simulink model "learjet"  (Simulink 6.3)
settings: Solver=ode4  StartTime=0.0  StopTime=100.0  FixedStep=0.1  RelTol=1e-3
values from neighbouring files (symbols this model uses):
  bref = 34    [learjet_iterate_trim_hood.m]    (also in learjet_iterate_trim_student.m; learjetstudent.m)
  cbar = 27.3    [hw5_714.m]    (also in hw6_714.m = 7; learjet_iterate_trim_hood.m = 7.04; learjet_iterate_trim_student.m = 7.04; learjetstudent.m = 7.04)
  CD0 = .0431    (= 0.0431)    [learjet_iterate_trim_hood.m]    (also in learjet_iterate_trim_student.m; learjetstudent.m = 0.1635)
  CD0BAR = .01867    (= 0.01867)    [learjet_iterate_trim_hood.m]    (also in learjet_iterate_trim_student.m; learjetstudent.m)
  CDA = 1.06    [learjet_iterate_trim_hood.m]    (also in learjet_iterate_trim_student.m; learjetstudent.m)
  CDDE = 0    [learjet_iterate_trim_hood.m]    (also in learjet_iterate_trim_student.m; learjetstudent.m)
  CDDETAB = 0    [learjet_iterate_trim_hood.m]    (also in learjet_iterate_trim_student.m; learjetstudent.m)
  CDK = .18824    (= 0.18824)    [learjet_iterate_trim_hood.m]    (also in learjet_iterate_trim_student.m; learjetstudent.m)
  CL0 = 1.2    [learjet_iterate_trim_hood.m]    (also in learjet_iterate_trim_student.m; learjetstudent.m)
  CLA = 5.04    [learjet_iterate_trim_hood.m]    (also in learjet_iterate_trim_student.m; learjetstudent.m)
  CLADOTHAT = 1.6    [learjet_iterate_trim_hood.m]    (also in learjet_iterate_trim_student.m; learjetstudent.m)
  CLDE = .40    (= 0.4)    [learjet_iterate_trim_hood.m]    (also in learjet_iterate_trim_student.m; learjetstudent.m)
  CLDETAB = CLDE/6.    (= 0.0666666666667)    [learjet_iterate_trim_hood.m]    (also in learjet_iterate_trim_student.m; learjetstudent.m)
  CLQHAT = 4.1    [learjet_iterate_trim_hood.m]    (also in learjet_iterate_trim_student.m; learjetstudent.m)
  CM0 = .047    (= 0.047)    [learjet_iterate_trim_hood.m]    (also in learjet_iterate_trim_student.m; learjetstudent.m)
  CMA = -.66    (= -0.66)    [learjet_iterate_trim_hood.m]    (also in learjet_iterate_trim_student.m; learjetstudent.m)
  CMADOTHAT = -5.0    (= -5)    [learjet_iterate_trim_hood.m]    (also in learjet_iterate_trim_student.m; learjetstudent.m)
  CMDE = -0.98    [learjet_iterate_trim_hood.m]    (also in learjet_iterate_trim_student.m; learjetstudent.m)
  CMDETAB = CMDE/6    (= -0.163333333333)    [learjet_iterate_trim_hood.m]    (also in learjet_iterate_trim_student.m; learjetstudent.m)
  CMQHAT = -13.5    [learjet_iterate_trim_hood.m]    (also in learjet_iterate_trim_student.m; learjetstudent.m)
  cosit = cos(it)    [learjet_iterate_trim_hood.m]    (also in learjet_iterate_trim_student.m; learjetstudent.m)
  detrim = dehat*(180/pi)    [learjet_iterate_trim_hood.m]    (also in learjet_iterate_trim_student.m; learjetstudent.m = 0)
  dPMdT = 0    [learjet_iterate_trim_hood.m]    (also in learjet_iterate_trim_student.m; learjetstudent.m)
  hic = 0    [learjet_iterate_trim_hood.m]    (also in learjet_iterate_trim_student.m; learjetstudent.m)
  inertia_matrix = [Ixxb 0 -Ixzb; 0 Iyyb 0;Ixzb 0 Izzb]    [learjet_iterate_trim_hood.m]    (also in learjet_iterate_trim_student.m; learjetstudent.m)
  mass = Wt/g    (= 403.726708075)    [learjet_iterate_trim_hood.m]    (also in learjet_iterate_trim_student.m; learjetstudent.m)
  phiic = 0    [learjet_iterate_trim_hood.m]    (also in learjet_iterate_trim_student.m; learjetstudent.m)
  psiic = 0    [learjet_iterate_trim_hood.m]    (also in learjet_iterate_trim_student.m; learjetstudent.m)
  sinit = sin(it)    [learjet_iterate_trim_hood.m]    (also in learjet_iterate_trim_student.m; learjetstudent.m)
  Sref = 232    [learjet_iterate_trim_hood.m]    (also in learjet_iterate_trim_student.m; learjetstudent.m)
  thetaic = alpha    [learjet_iterate_trim_hood.m]    (also in learjet_iterate_trim_student.m; learjetstudent.m = 0.0698131700798)
  thrust = thrusthat    [learjet_iterate_trim_hood.m]    (also in learjet_iterate_trim_student.m; learjetstudent.m = 1000)
  U1 = 100:50:400    [hw5_714.m]    (also in hw6_714.m = 170; learjet_iterate_trim_hood.m = 170; learjet_iterate_trim_student.m = 170; learjetstudent.m = 170)
  Uic = U1*cos(alpha)    [learjet_iterate_trim_hood.m]    (also in learjet_iterate_trim_student.m; learjetstudent.m)
  Vic = 0    [learjet_iterate_trim_hood.m]    (also in learjet_iterate_trim_student.m; learjetstudent.m)
  Wic = U1*sin(alpha)    [learjet_iterate_trim_hood.m]    (also in learjet_iterate_trim_student.m; learjetstudent.m)
  Wt = 13000    [learjet_iterate_trim_hood.m]    (also in learjet_iterate_trim_student.m; learjetstudent.m)
libraries: aerospace x7
settings Model: LastModifiedBy=jsteck  BufferReuse=off  StrictBusMsg=None
settings DataIOCC: SignalLoggingName=sigsOut
settings OptimizationCC: BooleanDataType=off  OptimizeBlockIOStorage=off  BufferReuse=off  ExpressionFolding=off  LocalBlockOutputs=off
settings DebuggingCC: SolverPrmCheckMsg=none
settings HardwareCC: TargetUnknown=on

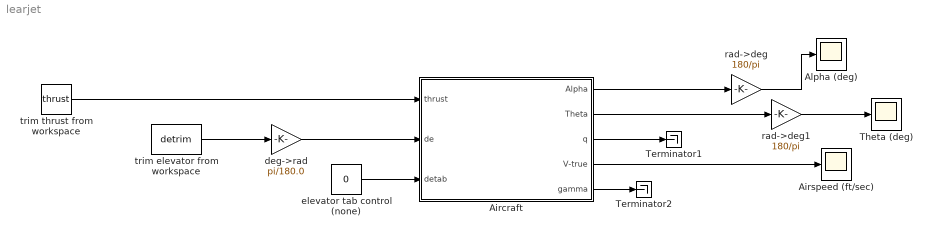
== system learjet ==
  Aircraft : Subsystem
  Airspeed (ft/sec) : Scope
      settings: TimeRange=100  YMin=100  YMax=200  SaveName=ScopeData4
  Alpha (deg) : Scope
      settings: TimeRange=100  YMin=0  YMax=8  SaveName=ScopeData3
  Terminator1 : Terminator
  Terminator2 : Terminator
  Theta (deg) : Scope
      settings: TimeRange=100  YMin=0  YMax=8  SaveName=ScopeData6
  deg->rad : Gain  Gain=pi/180.0  SaturateOnIntegerOverflow=on
  elevator tab control (none) : Constant  Value=0
  rad->deg : Gain  Gain=180/pi  SaturateOnIntegerOverflow=on
  rad->deg1 : Gain  Gain=180/pi  SaturateOnIntegerOverflow=on
  trim elevator from workspace : Constant  Value=detrim
  trim thrust from workspace : Constant  Value=thrust
  wires:
  elevator tab control (none)/1 -> Aircraft/3(detab)
  trim thrust from workspace/1 -> Aircraft/1(thrust)
  trim elevator from workspace/1 -> deg->rad/1
  Aircraft/1(Alpha) -> rad->deg/1
  Aircraft/4(V-true) -> Airspeed (ft/sec)/1
  Aircraft/2(Theta) -> rad->deg1/1
  Aircraft/3(q) -> Terminator1/1
  Aircraft/5(gamma) -> Terminator2/1
  deg->rad/1 -> Aircraft/2(de)
  rad->deg/1 -> Alpha (deg)/1
  rad->deg1/1 -> Theta (deg)/1

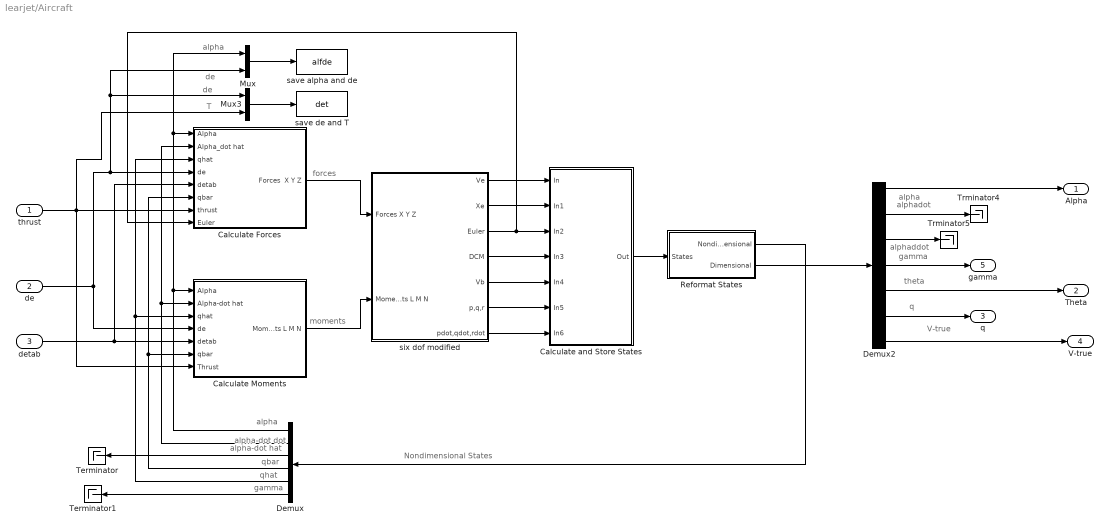
== system learjet/Aircraft ==
  note: Nondimensional States
  note: alpha
  note: alpha-dot hat
  note: gamma
  note: qbar
  note: forces
  note: moments
  note: de
  note: alpha
  note: de
  note: T
  note: alpha-dot dot
  note: qhat
  note: alpha
  note: alphadot
  note: alphaddot
  note: theta
  note: q
  note: gamma
  note: V-true
  thrust : Inport
  de : Inport  Port=2
  detab : Inport  Port=3
  Calculate Forces : Subsystem
  Calculate Moments : Subsystem
  Calculate and Store States : Subsystem
  Demux : Demux  Orientation=left  Outputs=6
  Demux2 : Demux  Outputs=7
  Mux : Mux  Inputs=2
  Mux3 : Mux  Inputs=2
  Reformat States : Subsystem
  Terminator : Terminator
  Terminator1 : Terminator
  Trminator4 : Terminator
  Trminator5 : Terminator
  save alpha and de : ToWorkspace  VariableName=alfde  SampleTime=-1  SaveFormat=Array
  save de and T : ToWorkspace  VariableName=det  SampleTime=-1  SaveFormat=Array
  six dof modified : Subsystem  AncestorBlock=aerospace/6DoF/Euler Angles  mask(6DoF Equations of Motion){xme_0=[0 0 hic], Vm_0=[Uic Vic Wic], eul_0=[phiic thetaic psiic], pm_0=[0 0 0], Mass=mass, Inertia=inertia_matrix}
      mask prompts: xme_0 "Initial position in inertial axes [Xe,Ye,Ze]:"; Vm_0 "Initial velocity in body axes [U,v,w]:"; eul_0 "Initial Euler orientation [roll, pitch, yaw]:"; pm_0 "Initial body rotation rates [p,q,r]:"; Inertia "Inertia matrix:"
      mask help: Integrates the 6 degrees of freedom equations of motion using an euler angle representation for the orientation of the body in space.
      mask Help:
      | <p>This block models a 6 degrees of freedom equations of motion for a rigid body using an euler angle representation.</p>
      | 
      | <pThe block inputs and outputs contain more than one signal as described below.</p>
      | 
      | <p><H4>Block Vector  Input - Forces X Y Z</H4>
      | <ul>
      |     <li>Forces on the body in X direction - X </li>
      |     <li>Forces on the body in Y direction - Y </li>
      |     <li>Forces on the body in Z direction - Z </li>
      | </ul>
      | </p>
      | <p><H4>Block Vector  Input - Moments L M N</H4>
      | <ul>
      |     <li>Moments on the body along X direction - L </li>
      |     <li>Moments on the body along Y direction - M </li>
      |     <li>Moments on the body along Z direction - N </li>
      | </ul>
      | </p>
      | <p><H4>Block Vector Output - Ve </H4>
      | <ul>
      |     <li>Translational velocity in X direction in Inertial coordinates </li>
      |     <li>Translational velocity in Y direction in Inertial coordinates </li>
      |     <li>Translational velocity in Z direction in Inertial coordinates </li>
      | </ul>
      | </p>
      | <p><H4>Block Vector Output - Xe </H4>
      | <ul>
      |     <li>Position in X direction in Inertial coordinates - Xe </li>
      |     <li>Position in Y direction in Inertial coordinates - Ye </li>
      |     <li>Position in Z direction in Inertial coordinates - Ze </li>
      | </ul>
      | </p>
      | <p><H4>Block Vector Output - Euler </H4>
      | <ul>
      |     <li>Phi ( radians )</li>
      |     <li>Theta ( radians )</li>
      |     <li>Psi ( radians )</li>
      | </ul>
      | </p>
      | <p><H4>Block Vector Output - DMC </H4>
      | <ul>
      |     <li>3x3 Directional Cosine Matrix</li>
      | </ul>
      | </p>
      | <p><H4>Block Vector Output - Vb</H4>
      | <ul>
      |     <li>Translational velocity in X direction in Body coordinates </li>
      |     <li>Translational velocity in Y direction in Body coordinates </li>
      |     <li>Translational velocity in Z direction in Body coordinates </li>
      | </ul>
      | </p>
      | <p><H4>Block Vector Output - p, q, r</H4>
      | <ul>
      |     <li>Roll rate - p ( radians/sec )</li>
      |     <li>Pitch rate - q ( radians/sec )</li>
      |     <li>Yaw rate - r ( radians/sec )</li>
      | </ul>
      | </p>
      | <p><H4>Block Vector Output - pdot, qdot, rdot</H4>
      | <ul>
      |     <li>Roll acceleration - pdot ( radians/sec^2 )</li>
      |     <li>Pitch acceleration - qdot ( radians/sec^2 )</li>
      |     <li>Yaw acceleration - rdot ( radians/sec^2 )</li>
      | </ul>
      | </p>
      mask Display: disp('Euler\nAngles')
  Alpha : Outport
  Theta : Outport  Port=2
  q : Outport  Port=3
  V-true : Outport  Port=4
  gamma : Outport  Port=5
  wires:
  six dof modified/4(DCM) -> Calculate and Store States/4(In3)
  six dof modified/3(Euler) -> Calculate Forces/8(Euler), Calculate and Store States/3(In2)
  six dof modified/1(Ve) -> Calculate and Store States/1(In)
  Calculate Moments/1(Moments L M N) -> six dof modified/2(Moments L M N)
  Demux/1 -> Calculate Moments/1(Alpha), Calculate Forces/1(Alpha), Mux/1
  Demux/2 -> Calculate Forces/2(Alpha_dot hat), Calculate Moments/2(Alpha-dot hat)
  detab/1 -> Calculate Moments/5(detab), Calculate Forces/5(detab)
  Mux/1 -> save alpha and de/1
  Reformat States/1(Nondimensional) -> Demux/1
  Mux3/1 -> save de and T/1
  six dof modified/2(Xe) -> Calculate and Store States/2(In1)
  Calculate Forces/1(Forces  X Y Z) -> six dof modified/1(Forces X Y Z)
  thrust/1 -> Mux3/2, Calculate Moments/7(Thrust), Calculate Forces/7(thrust)
  de/1 -> Mux/2, Mux3/1, Calculate Forces/4(de), Calculate Moments/4(de)
  Calculate and Store States/1(Out) -> Reformat States/1(States)
  Reformat States/2(Dimensional) -> Demux2/1
  Demux/3 -> Terminator/1
  Demux/4 -> Calculate Moments/6(qbar), Calculate Forces/6(qbar)
  Demux/5 -> Calculate Moments/3(qhat), Calculate Forces/3(qhat)
  Demux/6 -> Terminator1/1
  six dof modified/5(Vb) -> Calculate and Store States/5(In4)
  six dof modified/6(p,q,r) -> Calculate and Store States/6(In5)
  six dof modified/7(pdot,qdot,rdot) -> Calculate and Store States/7(In6)
  Demux2/6 -> q/1
  Demux2/1 -> Alpha/1
  Demux2/4 -> gamma/1
  Demux2/2 -> Trminator4/1
  Demux2/3 -> Trminator5/1
  Demux2/5 -> Theta/1
  Demux2/7 -> V-true/1

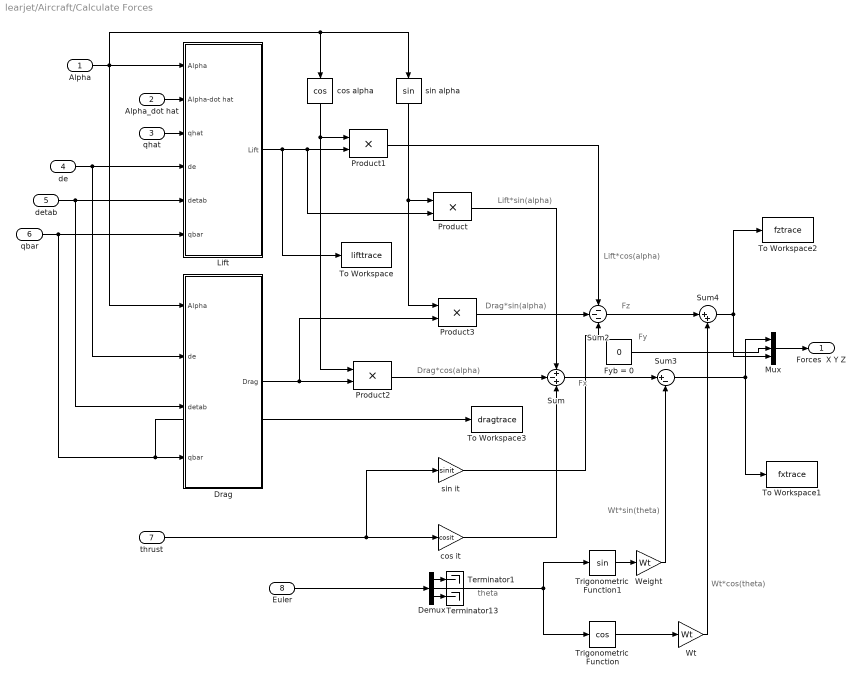
== system learjet/Aircraft/Calculate Forces ==
  note: Fz
  note: Fy
  note: Fx
  note: Lift*cos(alpha)
  note: Drag*sin(alpha)
  note: Drag*cos(alpha)
  note: Lift*sin(alpha)
  note: theta
  note: Wt*sin(theta)
  note: Wt*cos(theta)
  Alpha : Inport
  Alpha_dot hat : Inport  Port=2
  qhat : Inport  Port=3
  de : Inport  Port=4
  detab : Inport  Port=5
  qbar : Inport  Port=6
  thrust : Inport  Port=7
  Euler : Inport  Port=8
  Demux : Demux  Outputs=3
  Drag : Subsystem
  Fyb = 0 : Constant  Value=0
  Lift : Subsystem
  Mux : Mux  Inputs=3
  Product{,1..3} (4 alike) : Product  SaturateOnIntegerOverflow=on  InputSameDT=on
  Sum : Sum  Inputs=+-+  SaturateOnIntegerOverflow=on  InputSameDT=on
  Sum2 : Sum  Inputs=---  SaturateOnIntegerOverflow=on  InputSameDT=on
  Sum3 : Sum  Inputs=|+-  SaturateOnIntegerOverflow=on  InputSameDT=on
  Sum4 : Sum  Inputs=|++  SaturateOnIntegerOverflow=on  InputSameDT=on
  Terminator1 : Terminator
  Terminator13 : Terminator
  To Workspace : ToWorkspace  VariableName=lifttrace  SampleTime=-1  SaveFormat=Array
  To Workspace1 : ToWorkspace  VariableName=fxtrace  SampleTime=-1  SaveFormat=Array
  To Workspace2 : ToWorkspace  VariableName=fztrace  SampleTime=-1  SaveFormat=Array
  To Workspace3 : ToWorkspace  VariableName=dragtrace  SampleTime=-1  SaveFormat=Array
  Trigonometric Function : Trigonometry  Operator=cos
  Trigonometric Function1 : Trigonometry
  Weight : Gain  Gain=Wt  SaturateOnIntegerOverflow=on
  Wt : Gain  Gain=Wt  SaturateOnIntegerOverflow=on
  cos alpha : Trigonometry  Orientation=down  Operator=cos
  cos it : Gain  Gain=cosit  SaturateOnIntegerOverflow=on
  sin alpha : Trigonometry  Orientation=down
  sin it : Gain  Gain=sinit  SaturateOnIntegerOverflow=on
  Forces  X Y Z : Outport
  wires:
  Alpha/1 -> Lift/1(Alpha), Drag/1(Alpha), cos alpha/1, sin alpha/1
  de/1 -> Lift/4(de), Drag/2(de)
  detab/1 -> Lift/5(detab), Drag/3(detab)
  qbar/1 -> Lift/6(qbar), Drag/4(qbar), To Workspace3/1
  cos alpha/1 -> Product1/1, Product2/1
  Lift/1(Lift) -> Product1/2, Product/2, To Workspace/1
  sin alpha/1 -> Product/1, Product3/1
  Drag/1(Drag) -> Product2/2, Product3/2
  Product2/1 -> Sum/2
  Product/1 -> Sum/1
  cos it/1 -> Sum/3
  Product3/1 -> Sum2/2
  sin it/1 -> Sum2/3
  Fyb = 0/1 -> Mux/2
  Alpha_dot hat/1 -> Lift/2(Alpha-dot hat)
  qhat/1 -> Lift/3(qhat)
  thrust/1 -> cos it/1, sin it/1
  Product1/1 -> Sum2/1
  Euler/1 -> Demux/1
  Demux/2 -> Trigonometric Function1/1, Trigonometric Function/1
  Mux/1 -> Forces  X Y Z/1
  Trigonometric Function1/1 -> Weight/1
  Trigonometric Function/1 -> Wt/1
  Sum/1 -> Sum3/1
  Weight/1 -> Sum3/2
  Sum3/1 -> Mux/1, To Workspace1/1
  Sum2/1 -> Sum4/1
  Wt/1 -> Sum4/2
  Sum4/1 -> Mux/3, To Workspace2/1
  Demux/1 -> Terminator1/1
  Demux/3 -> Terminator13/1

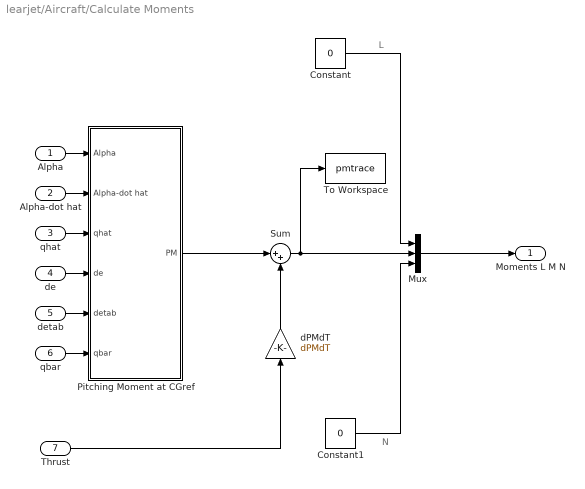
== system learjet/Aircraft/Calculate Moments ==
  note: L
  note: N
  Alpha : Inport
  Alpha-dot hat : Inport  Port=2
  qhat : Inport  Port=3
  de : Inport  Port=4
  detab : Inport  Port=5
  qbar : Inport  Port=6
  Thrust : Inport  Port=7
  Constant : Constant  Value=0
  Constant1 : Constant  Value=0
  Mux : Mux  Inputs=3
  Pitching Moment at CGref : Subsystem
  Sum : Sum  Inputs=|++  SaturateOnIntegerOverflow=on  InputSameDT=on
  To Workspace : ToWorkspace  VariableName=pmtrace  SampleTime=-1  SaveFormat=Array
  dPMdT : Gain  Orientation=up  Gain=dPMdT  SaturateOnIntegerOverflow=on
  Moments L M N : Outport
  wires:
  Constant/1 -> Mux/1
  Constant1/1 -> Mux/3
  Alpha/1 -> Pitching Moment at CGref/1(Alpha)
  Alpha-dot hat/1 -> Pitching Moment at CGref/2(Alpha-dot hat)
  qhat/1 -> Pitching Moment at CGref/3(qhat)
  Mux/1 -> Moments L M N/1
  de/1 -> Pitching Moment at CGref/4(de)
  detab/1 -> Pitching Moment at CGref/5(detab)
  qbar/1 -> Pitching Moment at CGref/6(qbar)
  Pitching Moment at CGref/1(PM) -> Sum/1
  dPMdT/1 -> Sum/2
  Sum/1 -> Mux/2, To Workspace/1
  Thrust/1 -> dPMdT/1

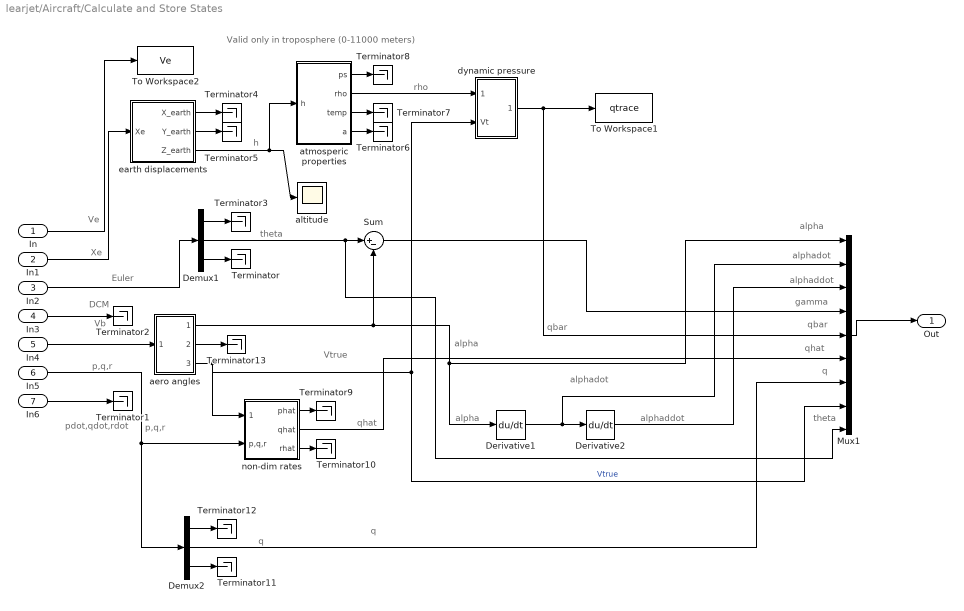
== system learjet/Aircraft/Calculate and Store States ==
  note: Euler
  note: DCM
  note: Vb
  note: p,q,r
  note: pdot,qdot,rdot
  note: Xe
  note: Ve
  note: Valid only in troposphere (0-11000 meters)
  note: alpha
  note: alphadot
  note: alphaddot
  note: qbar
  note: qhat
  note: gamma
  note: q
  note: theta
  note: q
  note: qhat
  note: p,q,r
  note: qbar
  note: Vtrue
  note: q
  note: rho
  note: h
  note: alpha
  note: alpha
  note: alphadot
  note: alphaddot
  note: theta
  In : Inport
  In1 : Inport  Port=2
  In2 : Inport  Port=3
  In3 : Inport  Port=4
  In4 : Inport  Port=5
  In5 : Inport  Port=6
  In6 : Inport  Port=7
  Demux1 : Demux  Outputs=3
  Demux2 : Demux  Outputs=3
  Derivative1 : Derivative
  Derivative2 : Derivative
  Mux1 : Mux  Inputs=9
  Sum : Sum  Inputs=|+-  SaturateOnIntegerOverflow=on  InputSameDT=on
  Terminator{,1..13} (14 alike) : Terminator
  To Workspace1 : ToWorkspace  VariableName=qtrace  SampleTime=-1  SaveFormat=Array
  To Workspace2 : ToWorkspace  VariableName=Ve  SampleTime=-1  SaveFormat=Array
  aero angles : Subsystem
  altitude : Scope
      settings: TimeRange=100  YMin=100  YMax=200  SaveName=ScopeData5
  atmosperic properties : Subsystem
  dynamic pressure : Subsystem
  earth displacements : Subsystem
  non-dim rates : Subsystem
  Out : Outport
  wires:
  In/1 -> To Workspace2/1
  In1/1 -> earth displacements/1(Xe)
  In4/1 -> aero angles/1(In1)
  In5/1 -> non-dim rates/2(p,q,r), Demux2/1
  In3/1 -> Terminator2/1
  In6/1 -> Terminator1/1
  In2/1 -> Demux1/1
  Demux1/3 -> Terminator/1
  Demux1/1 -> Terminator3/1
  Demux1/2 -> Sum/1, Mux1/9
  earth displacements/3(Z_earth) -> atmosperic properties/1(h), altitude/1
  earth displacements/1(X_earth) -> Terminator4/1
  earth displacements/2(Y_earth) -> Terminator5/1
  aero angles/3(Vtrue) -> non-dim rates/1(V true), Mux1/8, dynamic pressure/2(Vt)  "Vtrue"
  atmosperic properties/2(rho) -> dynamic pressure/1(rho)
  atmosperic properties/1(ps) -> Terminator8/1
  atmosperic properties/3(temp) -> Terminator7/1
  dynamic pressure/1(qbar) -> To Workspace1/1, Mux1/5
  Mux1/1 -> Out/1
  non-dim rates/2(qhat) -> Mux1/6
  non-dim rates/3(rhat) -> Terminator10/1
  non-dim rates/1(phat) -> Terminator9/1
  Demux2/3 -> Terminator11/1
  Demux2/2 -> Mux1/7
  Demux2/1 -> Terminator12/1
  aero angles/2(Beta) -> Terminator13/1
  aero angles/1(Alpha) -> Sum/2, Derivative1/1, Mux1/1
  Derivative2/1 -> Mux1/3
  Sum/1 -> Mux1/4
  Derivative1/1 -> Derivative2/1, Mux1/2
  atmosperic properties/4(a) -> Terminator6/1

== system learjet/Aircraft/Reformat States ==
  note: alpha
  note: alphadot
  note: alphaddot
  note: qbar
  note: qhat
  note: gamma
  note: q
  note: alpha
  note: alpha-dot hat
  note: qhat
  note: qbar
  note: alpha
  note: alphadot
  note: alphaddot
  note: theta
  note: q
  note: gamma
  note: alphaddot
  note: gamma
  note: theta
  States : Inport
  Demux1 : Demux  Outputs=9
  Mux1 : Mux  Inputs=6
  Mux2 : Mux  Inputs=7
  cbar/2U1 : Gain  Gain=cbar/(2*U1)  SaturateOnIntegerOverflow=on
  Nondimensional : Outport
  Dimensional : Outport  Port=2
  wires:
  States/1 -> Demux1/1
  Mux1/1 -> Nondimensional/1
  Mux2/1 -> Dimensional/1
  cbar/2U1/1 -> Mux1/2
  Demux1/7 -> Mux2/6
  Demux1/3 -> Mux2/3, Mux1/3
  Demux1/2 -> cbar/2U1/1, Mux2/2
  Demux1/1 -> Mux1/1, Mux2/1
  Demux1/4 -> Mux2/4, Mux1/6
  Demux1/8 -> Mux2/7  "Vtrue"
  Demux1/5 -> Mux1/4
  Demux1/6 -> Mux1/5
  Demux1/9 -> Mux2/5

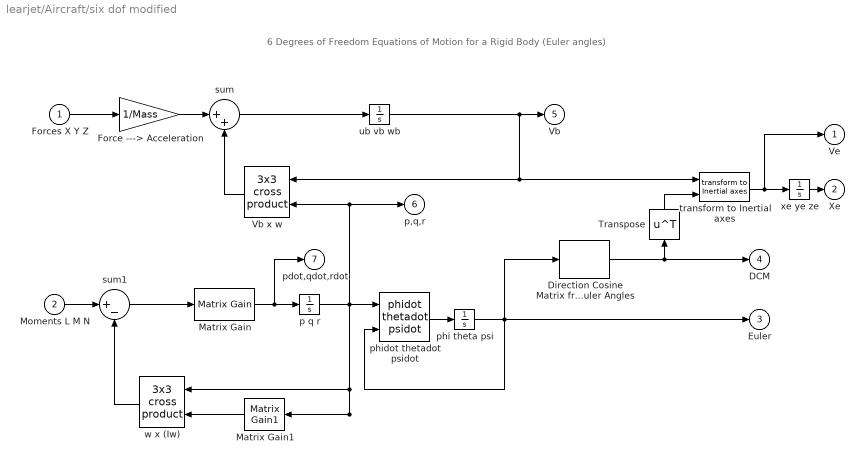
== system learjet/Aircraft/six dof modified ==
  note: 6 Degrees of Freedom Equations of Motion for a Rigid Body
      | (Euler angles)
  Forces X Y Z : Inport
  Moments L M N : Inport  Port=2
  Direction Cosine Matrix from Euler Angles : aerospace/Axes Transformations/Direction Cosine Matrix from Euler Angles
  Force ---> Acceleration : Gain  Gain=1/Mass  SaturateOnIntegerOverflow=on
  Matrix Gain : aerospace/6DoF/Euler Angles/Matrix Gain  MaskParam1=inv(Inertia)
  Matrix Gain1 : aerospace/6DoF/Euler Angles/Matrix Gain1  Orientation=left  MaskParam1=Inertia
  Transpose : Math  Orientation=up  Operator=transpose  SaturateOnIntegerOverflow=on
  Vb x w : aerospace/Axes Transformations/3x3 cross product  Orientation=left
  p q r : Integrator  InitialCondition=pm_0
  phi theta psi : Integrator  InitialCondition=eul_0
  phidot thetadot psidot : aerospace/6DoF/Euler Angles/phidot thetadot psidot
  sum : Sum  Inputs=|++  SaturateOnIntegerOverflow=on  InputSameDT=on
  sum1 : Sum  Inputs=|+-  SaturateOnIntegerOverflow=on  InputSameDT=on
  "transform to Inertial axes " : aerospace/6DoF/Euler Angles/transform to Inertial axes 
  ub vb wb : Integrator  InitialCondition=Vm_0
  w x (Iw) : aerospace/Axes Transformations/3x3 cross product  Orientation=left
  xe ye ze : Integrator  InitialCondition=xme_0
  Ve : Outport  InitialOutput=0
  Xe : Outport  Port=2  InitialOutput=0
  Euler : Outport  Port=3  InitialOutput=0
  DCM : Outport  Port=4  InitialOutput=0
  Vb : Outport  Port=5  InitialOutput=0
  p,q,r : Outport  Port=6  InitialOutput=0
  pdot,qdot,rdot : Outport  Port=7  InitialOutput=0
  wires:
  phidot thetadot psidot/1 -> phi theta psi/1
  phi theta psi/1 -> Euler/1, phidot thetadot psidot/2, Direction Cosine Matrix from Euler Angles/1
  ub vb wb/1 -> Vb/1, Vb x w/1, "transform to Inertial axes "/1
  sum/1 -> ub vb wb/1
  xe ye ze/1 -> Xe/1
  "transform to Inertial axes "/1 -> xe ye ze/1, Ve/1
  p q r/1 -> Vb x w/2, p,q,r/1, Matrix Gain1/1, phidot thetadot psidot/1, w x (Iw)/1
  sum1/1 -> Matrix Gain/1
  Moments L M N/1 -> sum1/1
  Matrix Gain1/1 -> w x (Iw)/2
  w x (Iw)/1 -> sum1/2
  Matrix Gain/1 -> p q r/1, pdot,qdot,rdot/1
  Forces X Y Z/1 -> Force ---> Acceleration/1
  Vb x w/1 -> sum/2
  Force ---> Acceleration/1 -> sum/1
  Direction Cosine Matrix from Euler Angles/1 -> Transpose/1, DCM/1
  Transpose/1 -> "transform to Inertial axes "/2

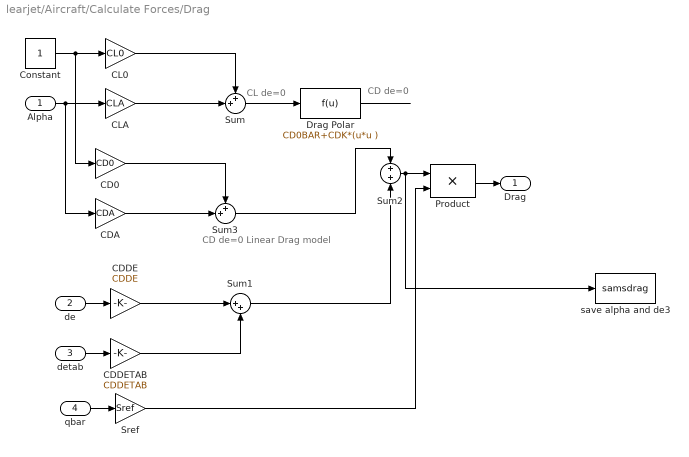
== system learjet/Aircraft/Calculate Forces/Drag ==
  note: CL de=0
  note: CD de=0
  note: CD de=0 Linear Drag model
  Alpha : Inport
  de : Inport  Port=2
  detab : Inport  Port=3
  qbar : Inport  Port=4
  CD0 : Gain  Gain=CD0  SaturateOnIntegerOverflow=on
  CDA : Gain  Gain=CDA  SaturateOnIntegerOverflow=on
  CDDE : Gain  Gain=CDDE  SaturateOnIntegerOverflow=on
  CDDETAB : Gain  Gain=CDDETAB  SaturateOnIntegerOverflow=on
  CL0 : Gain  Gain=CL0  SaturateOnIntegerOverflow=on
  CLA : Gain  Gain=CLA  SaturateOnIntegerOverflow=on
  Constant : Constant
  Drag Polar : Fcn  Expr=CD0BAR+CDK*(u*u )
  Product : Product  SaturateOnIntegerOverflow=on  InputSameDT=on
  Sref : Gain  Gain=Sref  SaturateOnIntegerOverflow=on
  Sum : Sum  Inputs=++|  SaturateOnIntegerOverflow=on  InputSameDT=on
  Sum1 : Sum  Inputs=|++  SaturateOnIntegerOverflow=on  InputSameDT=on
  Sum2 : Sum  Inputs=+|+  SaturateOnIntegerOverflow=on  InputSameDT=on
  Sum3 : Sum  Inputs=++|  SaturateOnIntegerOverflow=on  InputSameDT=on
  save alpha and de3 : ToWorkspace  VariableName=samsdrag  SampleTime=-1  SaveFormat=Array
  Drag : Outport
  wires:
  Constant/1 -> CL0/1, CD0/1
  CLA/1 -> Sum/2
  CL0/1 -> Sum/1
  Sum1/1 -> Sum2/2
  Sum2/1 -> Product/1, save alpha and de3/1
  Sref/1 -> Product/2
  Alpha/1 -> CLA/1, CDA/1
  Product/1 -> Drag/1
  de/1 -> CDDE/1
  detab/1 -> CDDETAB/1
  qbar/1 -> Sref/1
  CDDE/1 -> Sum1/1
  CDDETAB/1 -> Sum1/2
  Drag Polar/1 -> ?
  Sum/1 -> Drag Polar/1
  CDA/1 -> Sum3/2
  CD0/1 -> Sum3/1
  Sum3/1 -> Sum2/1

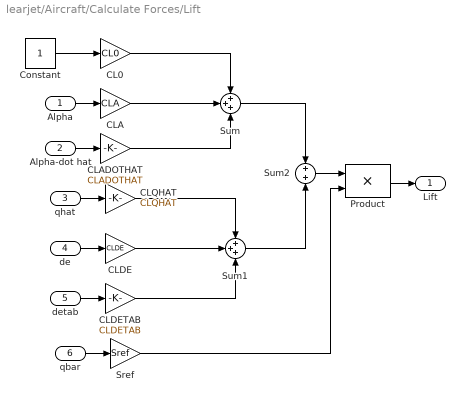
== system learjet/Aircraft/Calculate Forces/Lift ==
  Alpha : Inport
  Alpha-dot hat : Inport  Port=2
  qhat : Inport  Port=3
  de : Inport  Port=4
  detab : Inport  Port=5
  qbar : Inport  Port=6
  CL0 : Gain  Gain=CL0  SaturateOnIntegerOverflow=on
  CLA : Gain  Gain=CLA  SaturateOnIntegerOverflow=on
  CLADOTHAT : Gain  Gain=CLADOTHAT  SaturateOnIntegerOverflow=on
  CLDE : Gain  Gain=CLDE  SaturateOnIntegerOverflow=on
  CLDETAB : Gain  Gain=CLDETAB  SaturateOnIntegerOverflow=on
  CLQHAT : Gain  Gain=CLQHAT  SaturateOnIntegerOverflow=on
  Constant : Constant
  Product : Product  SaturateOnIntegerOverflow=on  InputSameDT=on
  Sref : Gain  Gain=Sref  SaturateOnIntegerOverflow=on
  Sum : Sum  Inputs=+++  SaturateOnIntegerOverflow=on  InputSameDT=on
  Sum1 : Sum  Inputs=+++  SaturateOnIntegerOverflow=on  InputSameDT=on
  Sum2 : Sum  Inputs=+|+  SaturateOnIntegerOverflow=on  InputSameDT=on
  Lift : Outport
  wires:
  Constant/1 -> CL0/1
  CLDE/1 -> Sum1/2
  CLA/1 -> Sum/2
  CL0/1 -> Sum/1
  CLADOTHAT/1 -> Sum/3
  CLQHAT/1 -> Sum1/1
  CLDETAB/1 -> Sum1/3
  Sum/1 -> Sum2/1
  Sum1/1 -> Sum2/2
  Sum2/1 -> Product/1
  Sref/1 -> Product/2
  Alpha/1 -> CLA/1
  Alpha-dot hat/1 -> CLADOTHAT/1
  Product/1 -> Lift/1
  qhat/1 -> CLQHAT/1
  de/1 -> CLDE/1
  detab/1 -> CLDETAB/1
  qbar/1 -> Sref/1

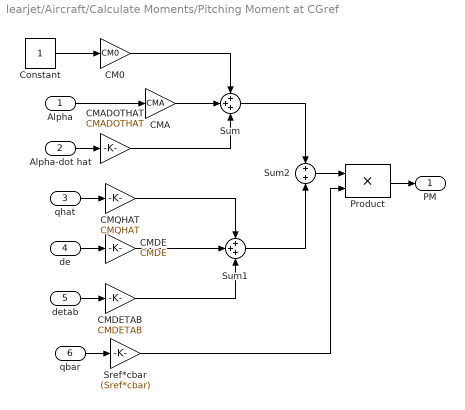
== system learjet/Aircraft/Calculate Moments/Pitching Moment at CGref ==
  Alpha : Inport
  Alpha-dot hat : Inport  Port=2
  qhat : Inport  Port=3
  de : Inport  Port=4
  detab : Inport  Port=5
  qbar : Inport  Port=6
  CM0 : Gain  Gain=CM0  SaturateOnIntegerOverflow=on
  CMA : Gain  Gain=CMA  SaturateOnIntegerOverflow=on
  CMADOTHAT : Gain  Gain=CMADOTHAT  SaturateOnIntegerOverflow=on
  CMDE : Gain  Gain=CMDE  SaturateOnIntegerOverflow=on
  CMDETAB : Gain  Gain=CMDETAB  SaturateOnIntegerOverflow=on
  CMQHAT : Gain  Gain=CMQHAT  SaturateOnIntegerOverflow=on
  Constant : Constant
  Product : Product  SaturateOnIntegerOverflow=on  InputSameDT=on
  Sref*cbar : Gain  Gain=(Sref*cbar)  SaturateOnIntegerOverflow=on
  Sum : Sum  Inputs=+++  SaturateOnIntegerOverflow=on  InputSameDT=on
  Sum1 : Sum  Inputs=+++  SaturateOnIntegerOverflow=on  InputSameDT=on
  Sum2 : Sum  Inputs=+|+  SaturateOnIntegerOverflow=on  InputSameDT=on
  PM : Outport
  wires:
  Constant/1 -> CM0/1
  CMDE/1 -> Sum1/2
  CMA/1 -> Sum/2
  CM0/1 -> Sum/1
  CMADOTHAT/1 -> Sum/3
  CMQHAT/1 -> Sum1/1
  CMDETAB/1 -> Sum1/3
  Sum/1 -> Sum2/1
  Sum1/1 -> Sum2/2
  Sum2/1 -> Product/1
  Sref*cbar/1 -> Product/2
  Alpha/1 -> CMA/1
  Alpha-dot hat/1 -> CMADOTHAT/1
  Product/1 -> PM/1
  qhat/1 -> CMQHAT/1
  de/1 -> CMDE/1
  detab/1 -> CMDETAB/1
  qbar/1 -> Sref*cbar/1

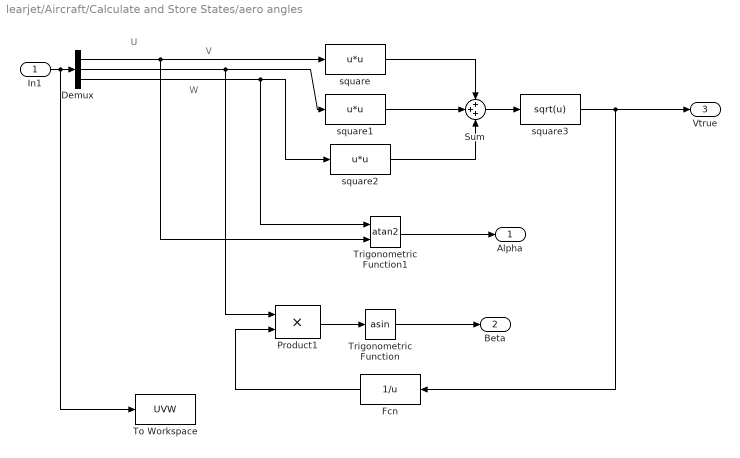
== system learjet/Aircraft/Calculate and Store States/aero angles ==
  note: U
  note: V
  note: W
  In1 : Inport
  Demux : Demux  Outputs=3
  Fcn : Fcn  Orientation=left  Expr=1/u
  Product1 : Product  SaturateOnIntegerOverflow=on  InputSameDT=on
  Sum : Sum  Inputs=+++  SaturateOnIntegerOverflow=on  InputSameDT=on
  To Workspace : ToWorkspace  VariableName=UVW  SampleTime=-1  SaveFormat=Array
  Trigonometric Function : Trigonometry  Operator=asin
  Trigonometric Function1 : Trigonometry  Operator=atan2
  square : Fcn  Expr=u*u
  square1 : Fcn  Expr=u*u
  square2 : Fcn  Expr=u*u
  square3 : Fcn  Expr=sqrt(u)
  Alpha : Outport
  Beta : Outport  Port=2
  Vtrue : Outport  Port=3
  wires:
  Demux/1 -> square/1, Trigonometric Function1/2
  Demux/2 -> Product1/1, square1/1
  Demux/3 -> square2/1, Trigonometric Function1/1
  In1/1 -> Demux/1, To Workspace/1
  Product1/1 -> Trigonometric Function/1
  square1/1 -> Sum/2
  square/1 -> Sum/1
  square2/1 -> Sum/3
  Sum/1 -> square3/1
  square3/1 -> Vtrue/1, Fcn/1
  Trigonometric Function/1 -> Beta/1
  Trigonometric Function1/1 -> Alpha/1
  Fcn/1 -> Product1/2

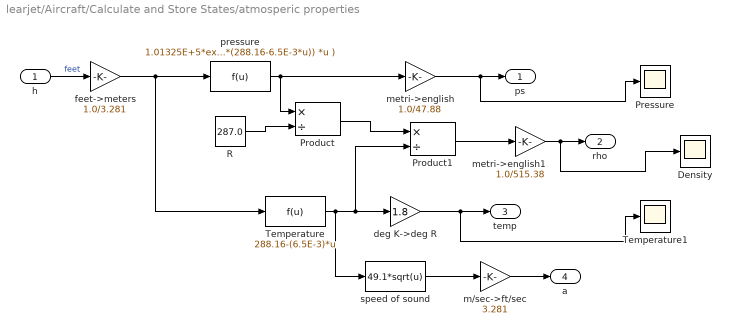
== system learjet/Aircraft/Calculate and Store States/atmosperic properties ==
  h : Inport
  Density : Scope
  Pressure : Scope
  Product : Product  Inputs=*/  SaturateOnIntegerOverflow=on
  Product1 : Product  Inputs=*/  SaturateOnIntegerOverflow=on
  R : Constant  Value=287.0
  Temperature : Fcn  Expr=288.16-(6.5E-3)*u
  Temperature1 : Scope
      settings: SaveName=ScopeData2
  deg K->deg R : Gain  Gain=1.8  SaturateOnIntegerOverflow=on
  feet->meters : Gain  Gain=1.0/3.281  SaturateOnIntegerOverflow=on
  m/sec->ft/sec : Gain  Gain=3.281  SaturateOnIntegerOverflow=on
  metri->english : Gain  Gain=1.0/47.88  SaturateOnIntegerOverflow=on
  metri->english1 : Gain  Gain=1.0/515.38  SaturateOnIntegerOverflow=on
  pressure : Fcn  Expr=1.01325E+5*exp( -9.81/(287*(288.16-6.5E-3*u)) *u )
  speed of sound : Fcn  Expr=49.1*sqrt(u)
  ps : Outport
  rho : Outport  Port=2
  temp : Outport  Port=3
  a : Outport  Port=4
  wires:
  pressure/1 -> metri->english/1, Product/1
  h/1 -> feet->meters/1  "feet"
  Product1/1 -> metri->english1/1
  Temperature/1 -> speed of sound/1, deg K->deg R/1, Product1/2
  speed of sound/1 -> m/sec->ft/sec/1
  feet->meters/1 -> Temperature/1, pressure/1
  metri->english/1 -> ps/1, Pressure/1
  metri->english1/1 -> rho/1, Density/1
  deg K->deg R/1 -> temp/1, Temperature1/1
  m/sec->ft/sec/1 -> a/1
  R/1 -> Product/2
  Product/1 -> Product1/1

== system learjet/Aircraft/Calculate and Store States/dynamic pressure ==
  rho : Inport
  Vt : Inport  Port=2
  Product : Product  Inputs=3  SaturateOnIntegerOverflow=on  InputSameDT=on
  half : Gain  Gain=1/2  SaturateOnIntegerOverflow=on
  qbar : Outport
  wires:
  Product/1 -> half/1
  Vt/1 -> Product/1, Product/2
  half/1 -> qbar/1
  rho/1 -> Product/3

== system learjet/Aircraft/Calculate and Store States/earth displacements ==
  Xe : Inport
  Demux : Demux  Outputs=3
  To Workspace : ToWorkspace  VariableName=xyz_earth  SampleTime=-1  SaveFormat=Array
  X_earth : Outport
  Y_earth : Outport  Port=2
  Z_earth : Outport  Port=3
  wires:
  Xe/1 -> To Workspace/1, Demux/1
  Demux/1 -> X_earth/1
  Demux/2 -> Y_earth/1
  Demux/3 -> Z_earth/1

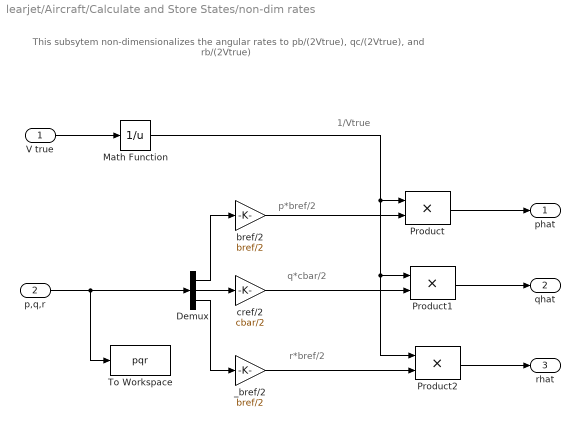
== system learjet/Aircraft/Calculate and Store States/non-dim rates ==
  note: p*bref/2
  note: q*cbar/2
  note: r*bref/2
  note: 1/Vtrue
  note: This subsytem non-dimensionalizes
      | the angular rates to pb/(2Vtrue),
      | qc/(2Vtrue), and rb/(2Vtrue)
  V true : Inport
  p,q,r : Inport  Port=2
  Demux : Demux  Outputs=3
  Math Function : Math  Operator=reciprocal  SaturateOnIntegerOverflow=on
  Product : Product  SaturateOnIntegerOverflow=on  InputSameDT=on
  Product1 : Product  SaturateOnIntegerOverflow=on  InputSameDT=on
  Product2 : Product  SaturateOnIntegerOverflow=on  InputSameDT=on
  To Workspace : ToWorkspace  VariableName=pqr  SampleTime=-1  SaveFormat=Array
  _bref/2 : Gain  Gain=bref/2  SaturateOnIntegerOverflow=on
  bref/2 : Gain  Gain=bref/2  SaturateOnIntegerOverflow=on
  cref/2 : Gain  Gain=cbar/2  SaturateOnIntegerOverflow=on
  phat : Outport
  qhat : Outport  Port=2
  rhat : Outport  Port=3
  wires:
  Demux/1 -> bref/2/1
  Demux/2 -> cref/2/1
  Demux/3 -> _bref/2/1
  p,q,r/1 -> Demux/1, To Workspace/1
  V true/1 -> Math Function/1
  bref/2/1 -> Product/2
  Product/1 -> phat/1
  cref/2/1 -> Product1/2
  Product1/1 -> qhat/1
  _bref/2/1 -> Product2/2
  Product2/1 -> rhat/1
  Math Function/1 -> Product/1, Product1/1, Product2/1
